simulink model "test_simulink2"  (R2013a)
settings: Solver=FixedStepDiscrete  StartTime=0.0  StopTime=200.0  RelTol=1e-3
values from neighbouring files (symbols this model uses):
  at = 1e-4    (= 0.0001)    [simu_ini.m]
  buff_size = frame_len    [simu2_ini.m]    (also in simu_ini.m = 11025)
  Fs = 22050    [simu_ini.m]
  rt = 50e-3    (= 0.05)    [simu_ini.m]
  samp_range_search = 100    [simu_ini.m]
  time_left = 2e-3    (= 0.002)    [simu_ini.m]
  time_right = 20e-3    (= 0.02)    [simu_ini.m]
undefined symbols (not defined in the file or in its folder): freq_left, freq_right, get, look_ahead_step, max_range, search_step, spectral_threshold_schiocco, thresh_bias, thresh_gain
libraries: simulink x4, dspsnks4 x3, dspmlti4 x1, dspsrcs4 x1, dspvision x1
settings Model: SimulationMode=accelerator  Creator=leonardo  LastModifiedBy=leonardo

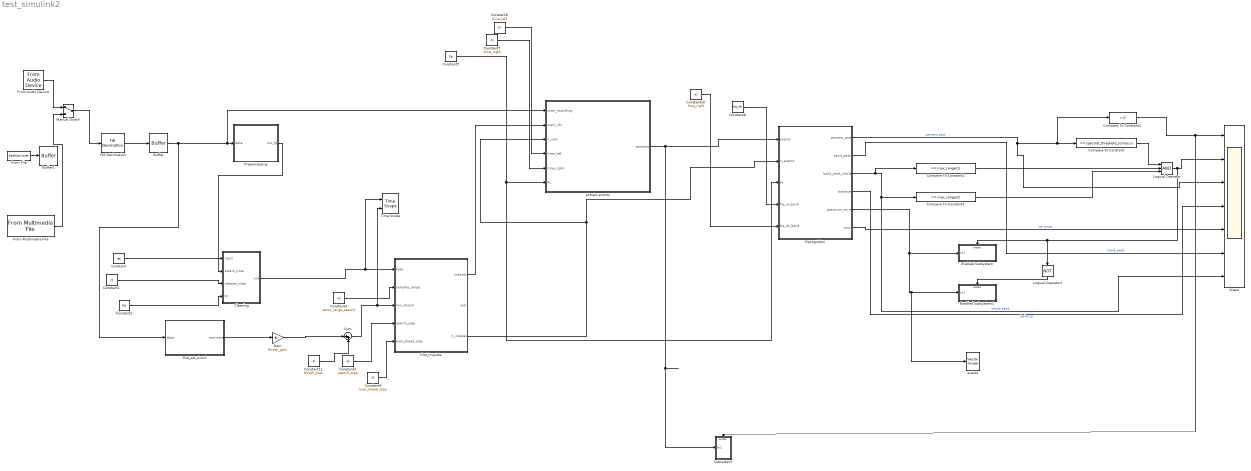
== system test_simulink2 ==
  Buffer : Buffer  N=buff_size  TreatMby1Signals=One channel
  Buffer1 : Buffer  N=2048  TreatMby1Signals=One channel
  Cleaning : MATLAB Function  TreatAsAtomicUnit=on
  Compare To Constant : simulink/Logic and Bit Operations/Compare To Constant  relop=>=  const=spectral_threshold_schiocco  OutDataTypeStr=boolean
  Compare To Constant1 : simulink/Logic and Bit Operations/Compare To Constant  relop=>  const=0  OutDataTypeStr=boolean
  Compare To Constant2 : simulink/Logic and Bit Operations/Compare To Constant  relop=>=  const=max_range(1)  OutDataTypeStr=boolean
  Compare To Constant3 : simulink/Logic and Bit Operations/Compare To Constant  relop=<=  const=max_range(2)  OutDataTypeStr=boolean
  Constant : Constant  Value=at
  Constant1 : Constant  Value=rt
  Constant10 : Constant  Value=freq_right
  Constant11 : Constant  Value=thresh_bias  VectorParams1D=off
  Constant2 : Constant  Value=Fs
  Constant3 : Constant  Value=search_step  VectorParams1D=off
  Constant4 : Constant  Value=samp_range_search
  Constant5 : Constant  Value=Fs
  Constant6 : Constant  Value=time_left
  Constant7 : Constant  Value=time_right
  Constant8 : Constant  Value=freq_left
  Constant9 : Constant  Value=look_ahead_step  VectorParams1D=off
  Enabled Subsystem : Subsystem  TreatAsAtomicUnit=on
  Enabled Subsystem1 : Subsystem  TreatAsAtomicUnit=on
  FIR Decimation : dspmlti4/FIR Decimation  h=fir1(35,0.4)  D=2  filtStruct=Direct form  framing=Enforce single-rate processing  inputOffset=0  outputBufInitCond=0  InputProcessing=Columns as channels (frame based)  firstCoeffDataTypeStr=Inherit: Same word length as input  firstCoeffLastDataTypeStr=Inherit: Same word length as input  firstCoeffMin=[]  firstCoeffMax=[]  outputDataTypeStr=Inherit: Same as accumulator  outputLastDataTypeStr=Inherit: Same as accumulator  outputMin=[]  outputMax=[]  roundingMode=Floor  overflowMode=off  FilterSource=Specify via dialog  FilterObject=Hm_firdecim
      settings: allowOverrides=off
  From Audio Device : dspsrcs4/From Audio Device  deviceName=Default  numChannels=1  sampleRate=44100  deviceDatatype=16-bit integer  autoBufferSize=on  bufferSize=4096  queueDuration=1.0  frameSize=2048  outputDatatype=single
  From File : FromFile  FileName=fashion.mat  SampleTime=1/44100
  From Multimedia File : dspvision/From Multimedia File  inputFilename=/home/leonardo/Ubuntu_home/leonardo/WCPYS/Impulse_recognition/snaps/Snap-claudio-1.m4a  loop=on  numPlays=inf  outputStreams=Audio only  videoDataType=single  audioDataType=double  inheritSampleTime=on  userDefinedSampleTime=1/30  noAudioOutput=off  isIntensityVideo=off  fourcc=RGB  colorVideoFormat=Separate color signals  outputEOF=off  dataOrg=Column-major  audioFrameSize=2048  computeAudioFrameSize=off  outSamplingMode=Frame based
  Gain : Gain  Gain=thresh_gain
  Logical Operator : Logic  Inputs=3  AllPortsSameDT=off  OutDataTypeStr=boolean
  Logical Operator1 : Logic  Operator=NOT  AllPortsSameDT=off  OutDataTypeStr=boolean
  Manual Switch : ManualSwitch
  Poe_est_simul : MATLAB Function  TreatAsAtomicUnit=on
  Preprocessing : MATLAB Function  TreatAsAtomicUnit=on
  Recognition : MATLAB Function  TreatAsAtomicUnit=on
  Snaps : Scope  NumInputPorts=7
      settings: YMin=0~0~0~0~0~1000~1000  YMax=1.5~1.5~1~2~1000~4000~10000
  Subsystem : Subsystem
  Sum : Sum  Inputs=|++
  Time Scope : TimeScope  NumInputPorts=2  DefaultConfigurationName=spbscopes.TimeScopeBlockCfg
      settings: CopyFcn=scopeextensions.ScopeBlock.callback(gcbh, 'onBlockCopy', gcbh);  DeleteFcn=scopeextensions.ScopeBlock.callback(gcbh, 'onBlockDelete');  PreSaveFcn=scopeextensions.ScopeBlock.callback(gcbh, 'onModelSave');  NameChangeFcn=scopeextensions.ScopeBlock.callback(gcbh, 'onBlockRename');  CloseFcn=scopeextensions.ScopeBlock.callback(gcbh, 'onBlockClose');  PreDeleteFcn=scopeextensions.ScopeBlock.callback(gcbh, 'onBlockPreDelete');
  events : dspsnks4/Vector Scope  ScopeProperties=on  Domain=User-defined  HorizSpan=1  DisplayProperties=off  AxisGrid=off  Memory=on  FrameNumber=on  AxisLegend=off  AxisZoom=off  OpenScopeAtSimStart=on  OpenScopeImmediately=off  FigPos=get(0,'defaultfigureposition')  AxisProperties=off  XUnits=Hertz  XRange=[0...Fs/2]  InheritXIncr=off  XIncr=1  XLabel=Frequency  XLimit=User-defined  XMin=0  XMax=256  XStart=0  YUnits=Magnitude  YLabel=Magnitude  LineProperties=off  XAxisParamsVer=6.9
      settings: YMin=0  YMax=1
  extract events : MATLAB Function  TreatAsAtomicUnit=on
  find_impulse : MATLAB Function  TreatAsAtomicUnit=on
  wires:
  Constant/1 -> Cleaning/2(attack_time)
  Constant1/1 -> Cleaning/3(release_time)
  Preprocessing/1(out_tg) -> Cleaning/1(input)
  Constant4/1 -> find_impulse/2(samples_range)
  Constant6/1 -> extract events/4(time_left)
  Constant7/1 -> extract events/5(time_right)
  find_impulse/1(indexes) -> extract events/2(main_idx)
  Buffer/1 -> Poe_est_simul/1(data), extract events/1(total_recording), Preprocessing/1(data)
  extract events/1(samples) -> Subsystem/1(In1), Recognition/1(events)
  find_impulse/3(n_indexes) -> Recognition/2(n_events), extract events/3(n_indx)
  FIR Decimation/1 -> Buffer/1
  Constant2/1 -> Cleaning/4(Fs)
  Constant5/1 -> Recognition/3(Fs), extract events/6(Fs)
  Constant8/1 -> Recognition/4(frq_sx_band)
  Constant10/1 -> Recognition/5(frq_dx_band)
  Cleaning/1(out) -> Time Scope/1, find_impulse/1(data)
  Recognition/1(percent_pow) -> Snaps/3, Compare To Constant1/1, Compare To Constant/1  "percent pow"
  Logical Operator/1 -> Enabled Subsystem/Enable, Logical Operator1/1, Snaps/2
  Compare To Constant/1 -> Logical Operator/1
  Compare To Constant2/1 -> Logical Operator/2
  Compare To Constant3/1 -> Logical Operator/3
  Constant3/1 -> find_impulse/4(search_step)
  Constant9/1 -> find_impulse/5(look_ahead_step)
  Gain/1 -> Sum/1
  Sum/1 -> Time Scope/2, find_impulse/3(min_thresh)
  Constant11/1 -> Sum/2
  Recognition/4(balance) -> Snaps/4  "balance"
  Recognition/6(vara) -> Snaps/5  "variance"
  Recognition/2(band_peak) -> Snaps/6  "band_peak"
  Logical Operator1/1 -> Enabled Subsystem1/Enable
  Recognition/3(band_peak_whole) -> Compare To Constant2/1, Compare To Constant3/1, Snaps/7  "whole peak"
  Poe_est_simul/1(estimate) -> Gain/1
  From Audio Device/1 -> Manual Switch/1
  Manual Switch/1 -> FIR Decimation/1
  From File/1 -> Buffer1/1
  Recognition/5(spectrum_norm) -> events/1, Enabled Subsystem1/1(In1), Enabled Subsystem/1(In1)
  From Multimedia File/1 -> Manual Switch/2
  Compare To Constant1/1 -> Subsystem/Enable, Snaps/1

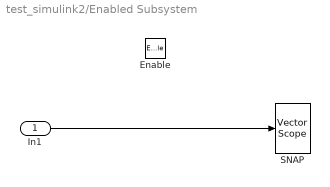
== system test_simulink2/Enabled Subsystem ==
  In1 : Inport
  Enable : EnablePort
  SNAP : dspsnks4/Vector Scope  ScopeProperties=on  Domain=User-defined  HorizSpan=1  DisplayProperties=off  AxisGrid=off  Memory=on  FrameNumber=on  AxisLegend=off  AxisZoom=off  OpenScopeAtSimStart=on  OpenScopeImmediately=off  FigPos=get(0,'defaultfigureposition')  AxisProperties=off  XUnits=Hertz  XRange=[0...Fs/2]  InheritXIncr=off  XIncr=1  XLabel=Frequency  XLimit=User-defined  XMin=0  XMax=256  XStart=0  YUnits=Magnitude  YLabel=Magnitude  LineProperties=off  XAxisParamsVer=6.9
      settings: YMin=0  YMax=1
  wires:
  In1/1 -> SNAP/1

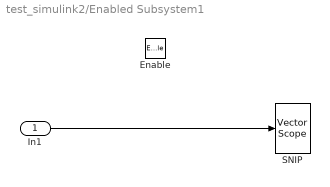
== system test_simulink2/Enabled Subsystem1 ==
  In1 : Inport
  Enable : EnablePort
  SNIP : dspsnks4/Vector Scope  ScopeProperties=on  Domain=User-defined  HorizSpan=1  DisplayProperties=off  AxisGrid=off  Memory=on  FrameNumber=on  AxisLegend=off  AxisZoom=off  OpenScopeAtSimStart=on  OpenScopeImmediately=off  FigPos=get(0,'defaultfigureposition')  AxisProperties=off  XUnits=Hertz  XRange=[0...Fs/2]  InheritXIncr=off  XIncr=1  XLabel=Frequency  XLimit=User-defined  XMin=0  XMax=256  XStart=0  YUnits=Magnitude  YLabel=Magnitude  LineProperties=off  XAxisParamsVer=6.9
      settings: YMin=0  YMax=1
  wires:
  In1/1 -> SNIP/1

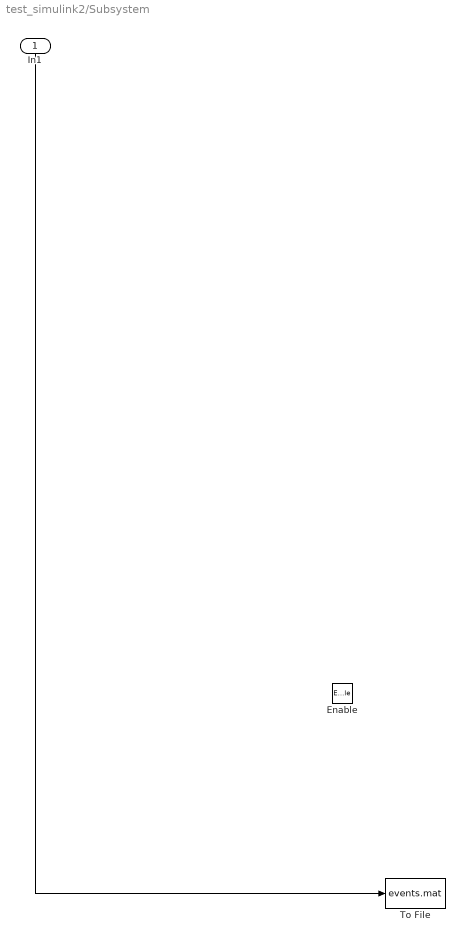
== system test_simulink2/Subsystem ==
  In1 : Inport
  Enable : EnablePort
  To File : ToFile  Filename=events.mat  MatrixName=data
  wires:
  In1/1 -> To File/1

== matlab function test_simulink2/Cleaning ==
  data: input input; out output; attack_time input; release_time input; Fs input
function out=xrms2(input,attack_time,release_time,Fs)

local_peak=abs(input(1));
len=length(input);
at = 1-exp(-2.2/(Fs*attack_time));
rt = 1-exp(-2.2/(Fs*release_time));
out=zeros(len,1);

out(1)=local_peak;

for i=2:len
    
    a=abs(input(i));
    
    if a > local_peak
        
        coeff = at;
        
    else
        
        coeff = rt;
    end
    
    local_peak = (1-coeff)*local_peak+coeff*a;
      
    out(i)=local_peak;

end

== matlab function test_simulink2/Preprocessing ==
  data: data input; out_tg output
function out_tg =detect_energy_threshold(data)


% Audio_info_T = struct('Expected_out',blanks(3),'Filename',blanks(64),'Samples',zeros(max_data_len,2),...
%     'Fs',0,'Nbits',0,'N_samples',0);
% 
% Audio_data=struct('Test_case',Audio_info_T);

% len = length(data);
% indexes = 

out_tg=teager_kaiser(data);

% indexes=find(out_tg>thresh);

end

function y = teager_kaiser(x)

% y = teager_kaiser(x) applies the Teager-Kaiser energy operator to
% input signal x.

x=x(:); % Setting x as a column vector

L = length(x);

y = x(2:L-1).^2-x(1:L-2).*x(3:L);
y = [y(1); y; y(L-2)]; % so that lenght(y)=length(x)

end

== matlab function test_simulink2/find_impulse ==
  data: data input; indexes output; samples_range input; min_thresh input; vals output; n_indexes output; search_step input; look_ahead_step input
function [indexes,vals,n_indexes]=find_local_max(data,samples_range,min_thresh,search_step,look_ahead_step)

len = length(data);
max_indexes = 4;
indexes=zeros(1,max_indexes);
vals=zeros(1,max_indexes);
k=1;
last_idx=0;
% max_sample_range=500;
% idx_l=zeros(1,max_sample_range);
% idx_r=zeros(1,max_sample_range);

for i = 3 : search_step : samples_range
    
%     idx_l(1,1:samples_range) = i-1:-1:i-samples_range;
%     idx_r(1,1:samples_range)  = i+1:i+samples_range;
skip = 0;
    if data(i)<=min_thresh(i) || min_thresh(i)<1e-10
        skip=1;
    else
         for j=i+look_ahead_step:look_ahead_step:i+samples_range
            a2 =  data(i)> data(j);
            if a2==0
                skip=1;
                break;
            end
         end
        if skip==0
            for j = i-look_ahead_step:-look_ahead_step:1 
                a1 =  data(i)> data(j);
                if a1==0
                    skip=1;
                    break;
                end
            end
        end
       
    end
 
    if skip==0

        indexes(k)=i;
        vals(k)=data(i);
        k=k+1;
    end
    
    last_idx = i;

end


for i = last_idx+search_step : search_step : len -samples_range -search_step
    
%     idx_l(1,1:samples_range) = i-1:-1:i-samples_range;
%     idx_r(1,1:samples_range)  = i+1:i+samples_range;
skip = 0;
    if data(i)<=min_thresh(i) || min_thresh(i)<1e-10
        skip=1;
    else
         for j=i+look_ahead_step:look_ahead_step:i+samples_range
            a2 =  data(i)> data(j);
            if a2==0
                skip=1;
                break;
            end
         end
        if skip==0
            for j = i-look_ahead_step:-look_ahead_step:i-samples_range 
                a1 =  data(i)> data(j);
                if a1==0
                    skip=1;
                    break;
                end
            end
        end
       
    end
 
    if skip==0

        indexes(k)=i;
        vals(k)=data(i);
        k=k+1;
    end
last_idx = i;
end

for i =  last_idx+search_step: search_step : len
    
%     idx_l(1,1:samples_range) = i-1:-1:i-samples_range;
%     idx_r(1,1:samples_range)  = i+1:i+samples_range;
skip = 0;
    if data(i)<=min_thresh(i) || min_thresh(i)<1e-10
        skip=1;
    else
         for j=i+look_ahead_step:look_ahead_step:len
            a2 =  data(i)> data(j);
            if a2==0
                skip=1;
                break;
            end
         end
        if skip==0
            for j = i-look_ahead_step:-look_ahead_step:i-samples_range 
                a1 =  data(i)> data(j);
                if a1==0
                    skip=1;
                    break;
                end
            end
        end
       
    end
 
    if skip==0

        indexes(k)=i;
        vals(k)=data(i);
        k=k+1;
    end

end
% last_idx = i;

[vals,sort_idx]=sort(vals,'descend');
indexes=indexes(sort_idx);
n_indexes=k-1;
end

== matlab function test_simulink2/extract events ==
  data: samples output; total_recording input; main_idx input; n_indx input; time_left input; time_right input; Fs input
function samples   = extract_events( total_recording,main_idx,n_indx,time_left,time_right,Fs)


max_idx=1;
actual_idx = n_indx;
% global Fs;
% n_indx=length(main_idx);
n_max_samples = ceil(30e-3*22050);%max_len*Fs;
 samples=zeros(n_max_samples,max_idx);
% sample_left=zeros(1,n_idx);
% sample_right=zeros(1,n_idx);
% samp_len=zeros(max_idx,1);

if n_indx>max_idx
    fprintf('too much indexes');
    actual_idx=max_idx;
end



for i=1:actual_idx
    
    sample_left = fix(main_idx(i)-time_left*Fs);
    sample_right = ceil(main_idx(i)+time_right*Fs);
    if sample_left<1
        sample_left=1;
    end
    if sample_right>length(total_recording)
        sample_right=length(total_recording);
    end
    extract_len=sample_right-sample_left+1;
%     samp_len(1:n_indx,i)=extract_len;
     samples(1:extract_len,i)=total_recording(sample_left:sample_right);
    
end




end

== matlab function test_simulink2/Poe_est_simul ==
  data: data input; estimate output
function estimate = pow_est(data)
%#codegen

n_slots = 2;
len = length(data);
j=0;
parzial_sum=single(0);
len_slot=fix(len/n_slots);
estimate = zeros(len,1);

while j<n_slots
    for i=1:len_slot
        parzial_sum = parzial_sum + data(j*len_slot+i)^2;
    end
    idxs = j*len_slot+1:(j+1)*len_slot;
    estimate(idxs) = parzial_sum/len_slot;
    parzial_sum=single(0);
    j=j+1;   
end

== matlab function test_simulink2/Recognition ==
  data: events input; percent_pow output; n_events input; Fs input; frq_sx_band input; frq_dx_band input; band_peak output; band_peak_whole output; balance output; spectrum_norm output; vara output
function [percent_pow,band_peak,band_peak_whole,balance,spectrum_norm,vara] = snap_recognition(events,n_events,Fs,frq_sx_band,frq_dx_band)



len_fft=512;


freq_step=Fs/(len_fft-1);
actual_events = n_events;

sx_bin_b2=round(frq_sx_band/freq_step)+1;
dx_bin_b2=round(frq_dx_band/freq_step)+1;
sel_len=dx_bin_b2-sx_bin_b2+1;
max_events=1;
 percent_pow=zeros(1,max_events);
 sel_pow2=zeros(1,max_events);
 tot_pow=zeros(1,max_events);
 spectrum=zeros(max_events,len_fft);
 
 bin_peak=zeros(1,max_events);
band_peak=zeros(1,max_events);
bin_peak_whole=zeros(1,max_events);
band_peak_whole=zeros(1,max_events);
max_peak=zeros(1,max_events);
max_peak_whole=zeros(1,max_events);
vara=zeros(1,max_events);
balance=zeros(1,max_events);
bal_range = round(500/freq_step)+1;
whole_pow_spec=zeros(len_fft/2,max_events);
 spectrum_norm=zeros(len_fft/2,max_events);
sel_pow_spec=zeros(max_events,len_fft/2);
% fft_axe=0:freq_step:Fs;
if n_events>max_events
    fprintf('too much events\n');
    actual_events=max_events;
end
% percent_pow1=0;
% percent_pow2=0;

     for i=1:actual_events
            fff = fft(events(1:len_fft,i));
          spectrum(i,:) = real(fff).^2+imag(fff).^2;
          spectrum(i,1:3) = 0;
          whole_pow_spec(:,i) = spectrum(i,1:len_fft/2);
          sel_pow_spec(i,1:sel_len) = spectrum(i,sx_bin_b2:dx_bin_b2);
        tot_pow(i) = sum(whole_pow_spec(:,i));
%         sel_pow1 = sum(spectrum(i,sx_bin_b1:dx_bin_b1));
        sel_pow2(i) = sum(sel_pow_spec(i,1:sel_len));
         vara(i)=var(sel_pow_spec(i,1:sel_len));
%         percent_pow(1,i)=sel_pow1/tot_pow;
        percent_pow(i)=sel_pow2(i)/tot_pow(i);
        
        [max_peak(i),bin_peak(i)]=max(sel_pow_spec);
         peak_idx = sx_bin_b2+bin_peak(i);
         band_peak(i)=(peak_idx-1)*freq_step;
         bal_right = peak_idx+bal_range;
         bal_left = peak_idx-bal_range;
         rp = sum(spectrum(i,peak_idx:1:bal_right));
         lp = sum(spectrum(i,peak_idx:-1:bal_left));
         balance(i)= rp/lp;
         [max_peak_whole(i),bin_peak_whole(i)]=max(whole_pow_spec(:,i));
         peak_idx_whole = bin_peak_whole(i);
         band_peak_whole(i)=(peak_idx_whole-1)*freq_step;
         max_pow = max_peak_whole(i);
         spectrum_norm(:,i)=whole_pow_spec(:,i)/max_pow;
     end
